simulink model "kamerol"  (R2021b)
settings: Solver=VariableStepAuto  StartTime=0.0  StopTime=10.0  RelTol=1e-3
undefined symbols (not defined in the file): admireDB
libraries: simulink_extras x104, simulink x24, sharedutil x1
(part 1 of 14)
settings Model: Creator=mehme  LastModifiedBy=mehme

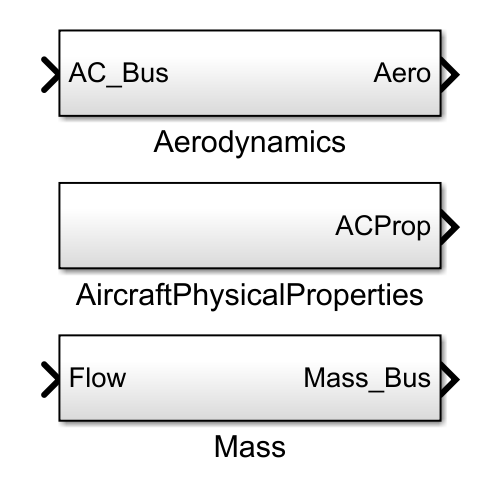
[thumbnail: Simulink's stored preview of the top-level diagram]
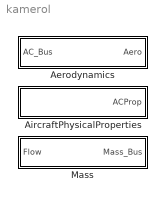
== system kamerol ==
  Aerodynamics : Subsystem
  AircraftPhysicalProperties : Subsystem
  Mass : Subsystem

== system kamerol/Aerodynamics ==
  AC_Bus : Inport
  Bus Creator1 : BusCreator  Inputs=12
  CentripetalForceCoefficient : Subsystem
  Interface : Subsystem
  NormalForceCoefficient : Subsystem
  PitchMomentCoefficient : Subsystem
  RollMomentCoefficient : Subsystem
  Subsystem : Subsystem
  TangentialForceCoefficient : Subsystem
  YawMomentCoefficient : Subsystem
  Aero : Outport
  wires:
  AC_Bus/1 -> Subsystem/7(AC_Bus), Interface/1(AC_Bus)  "AeroIn_Bus"
  PitchMomentCoefficient/1(Cpmtot) -> Subsystem/5(cpm), Bus Creator1/5  "pitchMomentCoeff_nd"
  NormalForceCoefficient/1(Cntot) -> Subsystem/3(cn), Bus Creator1/3  "normalForceCoeff_nd"
  TangentialForceCoefficient/1(Cttot) -> Bus Creator1/1, Subsystem/1(ct)  "tangentialForceCoeff_nd"
  Bus Creator1/1 -> Aero/1  "Aero_Bus"
  Interface/1(AeroIn_Bus) -> TangentialForceCoefficient/1(AeroIn_Bus), CentripetalForceCoefficient/1(AeroIn_Bus), NormalForceCoefficient/1(AeroIn_Bus), RollMomentCoefficient/1(AeroIn_Bus), YawMomentCoefficient/1(AeroIn_Bus), PitchMomentCoefficient/1(AeroIn_Bus)  "AeroIn_Bus"
  Subsystem/1(aeroForceBodyX_N) -> Bus Creator1/7  "aeroForceBodyX_N"
  Subsystem/2(aeroForceBodyY_N) -> Bus Creator1/8  "aeroForceBodyY_N"
  Subsystem/3(aeroForceBodyZ_N) -> Bus Creator1/9  "aeroForceBodyZ_N"
  Subsystem/4(aeroMomentBodyX_N) -> Bus Creator1/10  "aeroMomentBodyX_N"
  Subsystem/5(aeroMomentBodyY_N) -> Bus Creator1/11  "aeroMomentBodyY_N"
  Subsystem/6(aeroMomentBodyZ_N) -> Bus Creator1/12  "aeroMomentBodyZ_N"
  CentripetalForceCoefficient/1(Cctot) -> Subsystem/2(cc), Bus Creator1/2  "centripetalForceCoeff_nd"
  RollMomentCoefficient/1(Crmtot) -> Subsystem/4(crm), Bus Creator1/4  "rollMomentCoeff_nd"
  YawMomentCoefficient/1(Cymtot) -> Subsystem/6(cym), Bus Creator1/6  "yawMomentCoeff_nd"

== system kamerol/AircraftPhysicalProperties ==
  Bus Creator : BusCreator  Inputs=19
  EngineOffsetY_m : Constant  Value=0
  EngineOffsetZ_m : Constant  Value=-0.15
  ReferenceAreaCanard_m2 : Constant  Value=3.20
  ReferenceAreaInboardElevon_m2 : Constant  Value=1.2
  ReferenceAreaInboardLEF_m2 : Constant  Value=0.45
  ReferenceAreaOutboardElevon_m2 : Constant  Value=1.35
  ReferenceAreaOutboardLEF_m : Constant  Value=0.45
  ReferenceAreaRudder_m2 : Constant  Value=0.80
  ReferenceArea_m2 : Constant  Value=45
  ReferenceChordCanard_m : Constant  Value=1.30
  ReferenceChordInboardElevon_m : Constant  Value=0.95
  ReferenceChordInboardLEF_m : Constant  Value=0.40
  ReferenceChordOutboardElevon_m : Constant  Value=0.68
  ReferenceChordOutboardLEF_m : Constant  Value=0.35
  ReferenceChordRudder_m : Constant  Value=0.60
  ReferenceChord_m : Constant  Value=5.2
  ReferenceLengthAirbrake_m : Constant  Value=1.10
  ReferenceSpanCanard_m : Constant  Value=2.60
  ReferenceSpan_m : Constant  Value=10
  ACProp : Outport
  wires:
  ReferenceArea_m2/1 -> Bus Creator/1  "referenceArea_m2"
  ReferenceChord_m/1 -> Bus Creator/2  "referenceChord_m"
  ReferenceSpan_m/1 -> Bus Creator/3  "referenceSpan_m"
  ReferenceAreaInboardElevon_m2/1 -> Bus Creator/4  "referenceAreaInboardElevon_m2"
  ReferenceChordInboardElevon_m/1 -> Bus Creator/5  "referenceChordInboardElevon_m"
  ReferenceAreaOutboardElevon_m2/1 -> Bus Creator/6  "referenceAreaOutboardElevon_m2"
  ReferenceChordOutboardElevon_m/1 -> Bus Creator/7  "referenceChordOutboardElevon_m"
  ReferenceAreaInboardLEF_m2/1 -> Bus Creator/8  "referenceAreaInboardLEF_m2"
  ReferenceChordInboardLEF_m/1 -> Bus Creator/9  "referenceChordInboardLEF_m"
  ReferenceAreaOutboardLEF_m/1 -> Bus Creator/10  "referenceAreaOutboardLEF_m"
  ReferenceChordOutboardLEF_m/1 -> Bus Creator/11  "referenceChordOutboardLEF_m"
  ReferenceAreaRudder_m2/1 -> Bus Creator/12  "referenceAreaRudder_m2"
  ReferenceChordRudder_m/1 -> Bus Creator/13  "referenceChordRudder_m"
  ReferenceLengthAirbrake_m/1 -> Bus Creator/14  "referenceLengthAirbrake_m"
  ReferenceAreaCanard_m2/1 -> Bus Creator/15  "referenceAreaCanard_m2"
  ReferenceChordCanard_m/1 -> Bus Creator/16  "referenceChordCanard_m"
  ReferenceSpanCanard_m/1 -> Bus Creator/17  "referenceSpanCanard_m"
  Bus Creator/1 -> ACProp/1  "AC_Bus"
  EngineOffsetY_m/1 -> Bus Creator/18  "engineOffsetY_m"
  EngineOffsetZ_m/1 -> Bus Creator/19  "engineOffsetZ_m"

== system kamerol/Mass ==
  Flow : Inport
  Bus Creator1 : BusCreator  Inputs=12
  Bus Selector : BusSelector  OutputSignals=DCM_Bus.dcmNED2Body
  Constant : Constant  Value=9.8065
  Constant1 : Constant  Value=0
  Constant3 : Constant  Value=0
  Demux : Demux  Outputs=3
  Inertia : Subsystem
  Matrix Multiply : Product  Multiplication=Matrix(*)
  Mux : Mux  Inputs=3
  Product : Product
  "mass " : Constant  Value=9100
  Mass_Bus : Outport
  wires:
  Bus Creator1/1 -> Mass_Bus/1  "MassBuss"
  Demux/1 -> Bus Creator1/8  "gravForceBodyX_N"
  Demux/2 -> Bus Creator1/9  "gravForceBodyY_N"
  Demux/3 -> Bus Creator1/10  "gravForceBodyZ_N"
  Constant3/1 -> Bus Creator1/11  "centerOfGravityBodyX_pct"
  "mass "/1 -> Bus Creator1/12, Product/2  "mass_kg"
  Flow/1 -> Bus Selector/1
  Constant/1 -> Product/1
  Bus Selector/1 -> Matrix Multiply/1  "<dcmNED2Body>"
  Constant1/1 -> Mux/2, Mux/1
  Product/1 -> Mux/3
  Matrix Multiply/1 -> Demux/1
  Mux/1 -> Matrix Multiply/2
  Inertia/1(InertiaTensor) -> Bus Creator1/1
  Inertia/2(inertiaIx_kgpm2) -> Bus Creator1/2
  Inertia/3(inertiaIy_kgpm2) -> Bus Creator1/3
  Inertia/4(inertiaIz_kgpm2) -> Bus Creator1/4
  Inertia/5(inertiaIxy_kgpm2) -> Bus Creator1/5
  Inertia/6(inertiaIxz_kgpm2) -> Bus Creator1/6
  Inertia/7(inertiaIyz_kgpm2) -> Bus Creator1/7

== system kamerol/Aerodynamics/CentripetalForceCoefficient ==
  AeroIn_Bus : Inport
  Bus Selector : BusSelector  OutputSignals=mach_nd
  MachRegion1 : Subsystem
  MachRegion2 : Subsystem
  MachRegion3 : Subsystem
  MachRegion4 : Subsystem
  Subsystem : Subsystem
  Cctot : Outport
  wires:
  Subsystem/1(Cctot) -> Cctot/1
  MachRegion3/1(cctot) -> Subsystem/4(CctotMR3)
  MachRegion2/1(cctot) -> Subsystem/3(CctotMR2)
  MachRegion4/1(cttot) -> Subsystem/5(CctotMR4)
  Bus Selector/1 -> Subsystem/1(mach_nd)  "<mach_nd>"
  AeroIn_Bus/1 -> MachRegion2/1(AeroIn_Bus), MachRegion3/1(AeroIn_Bus), MachRegion4/1(AeroIn_Bus), MachRegion1/1(AeroIn_Bus), Bus Selector/1
  MachRegion1/1(cctot) -> Subsystem/2(CctotMR1)

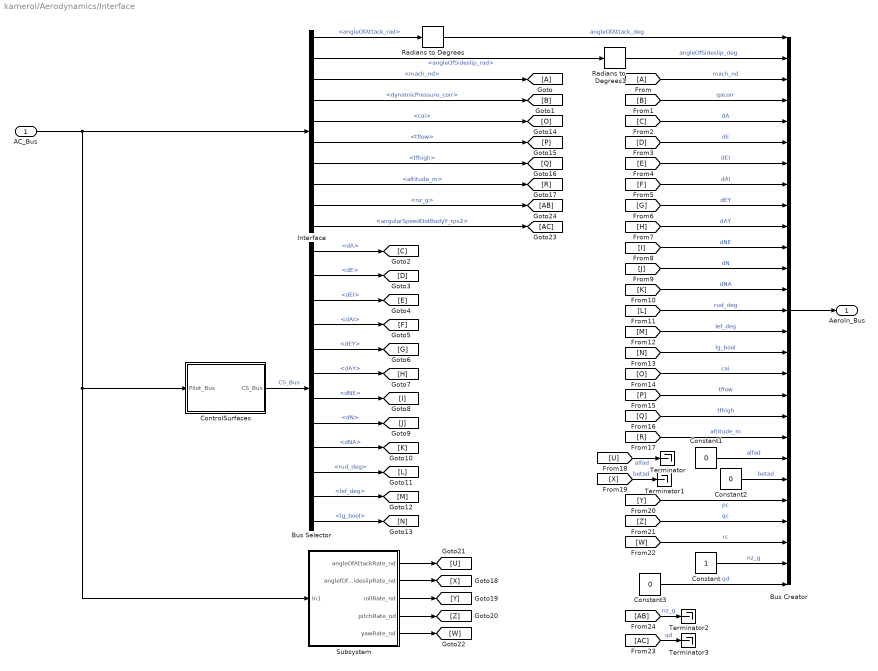
== system kamerol/Aerodynamics/Interface ==
  AC_Bus : Inport
  Bus Creator : BusCreator  Inputs=27
  Bus Selector : BusSelector  OutputSignals=dA,dE,dEI,dAI,dEY,dAY,dNE,dN,dNA,rud_deg,lef_deg,lg_bool
  Constant : Constant
  Constant1 : Constant  Value=0
  Constant2 : Constant  Value=0
  Constant3 : Constant  Value=0
  ControlSurfaces : Subsystem
  Interface : BusSelector  OutputSignals=EOM_Bus.angleOfAttack_rad,EOM_Bus.angleOfSideslip_rad,Env_Bus.mach_nd,Env_Bus.dynamicPressure_corr,Misc_Bus.cai,Env_Bus.tflow,Env_Bus.tfhigh,EOM_Bus.altitude_m,EOM_Bus.nz_g,EOM_Bus.angularSpeedDotBodyY_rps2
  Radians to Degrees : simulink_extras/Transformations/Radians to Degrees
  Radians to Degrees1 : simulink_extras/Transformations/Radians to Degrees
  Subsystem : Subsystem
  Terminator{,1..3} (4 alike) : Terminator
  AeroIn_Bus : Outport
  wires:
  AC_Bus/1 -> Subsystem/1(In1), ControlSurfaces/1(Pilot_Bus), Interface/1
  Bus Creator/1 -> AeroIn_Bus/1
  Interface/1 -> Radians to Degrees/1  "<angleOfAttack_rad>"
  Interface/2 -> Radians to Degrees1/1  "<angleOfSideslip_rad>"
  Radians to Degrees/1 -> Bus Creator/1  "angleOfAttack_deg"
  Radians to Degrees1/1 -> Bus Creator/2  "angleOfSideslip_deg"
  Interface/3 -> [A]  "<mach_nd>"
  [A] -> Bus Creator/3  "mach_nd"
  [B] -> Bus Creator/4  "qacorr"
  Interface/4 -> [B]  "<dynamicPressure_corr>"
  Interface/5 -> [O]  "<cai>"
  Interface/6 -> [P]  "<tflow>"
  Interface/7 -> [Q]  "<tfhigh>"
  Interface/8 -> [R]  "<altitude_m>"
  [C] -> Bus Creator/5  "dA"
  [D] -> Bus Creator/6  "dE"
  [E] -> Bus Creator/7  "dEI"
  [N] -> Bus Creator/16  "lg_bool"
  [F] -> Bus Creator/8  "dAI"
  [R] -> Bus Creator/20  "altitude_m"
  [O] -> Bus Creator/17  "cai"
  Constant1/1 -> Bus Creator/21  "alfad"
  Constant2/1 -> Bus Creator/22  "betad"
  [G] -> Bus Creator/9  "dEY"
  [H] -> Bus Creator/10  "dAY"
  [K] -> Bus Creator/13  "dNA"
  [L] -> Bus Creator/14  "rud_deg"
  [I] -> Bus Creator/11  "dNE"
  [J] -> Bus Creator/12  "dN"
  [M] -> Bus Creator/15  "lef_deg"
  [W] -> Bus Creator/25  "rc"
  [Q] -> Bus Creator/19  "tfhigh"
  [P] -> Bus Creator/18  "tflow"
  [Y] -> Bus Creator/23  "pc"
  [Z] -> Bus Creator/24  "qc"
  Constant/1 -> Bus Creator/26  "nz_g"
  Interface/9 -> [AB]  "<nz_g>"
  Interface/10 -> [AC]  "<angularSpeedDotBodyY_rps2>"
  Constant3/1 -> Bus Creator/27  "qd"
  Subsystem/2(anglefOfSideslipRate_nd) -> [X]
  Subsystem/1(angleOfAttackRate_nd) -> [U]
  Subsystem/3(rollRate_nd) -> [Y]
  Subsystem/4(pitchRate_nd) -> [Z]
  Subsystem/5(yawRate_nd) -> [W]
  [U] -> Terminator/1  "alfad"
  [X] -> Terminator1/1  "betad"
  [AB] -> Terminator2/1  "nz_g"
  [AC] -> Terminator3/1  "qd"
  ControlSurfaces/1(CS_Bus) -> Bus Selector/1  "CS_Bus"
  Bus Selector/1 -> [C]  "<dA>"
  Bus Selector/2 -> [D]  "<dE>"
  Bus Selector/3 -> [E]  "<dEI>"
  Bus Selector/4 -> [F]  "<dAI>"
  Bus Selector/5 -> [G]  "<dEY>"
  Bus Selector/6 -> [H]  "<dAY>"
  Bus Selector/7 -> [I]  "<dNE>"
  Bus Selector/8 -> [J]  "<dN>"
  Bus Selector/9 -> [K]  "<dNA>"
  Bus Selector/10 -> [L]  "<rud_deg>"
  Bus Selector/11 -> [M]  "<lef_deg>"
  Bus Selector/12 -> [N]  "<lg_bool>"

== system kamerol/Aerodynamics/NormalForceCoefficient ==
  AeroIn_Bus : Inport
  Bus Selector : BusSelector  OutputSignals=mach_nd
  MachRegion1 : Subsystem
  MachRegion2 : Subsystem
  MachRegion3 : Subsystem
  Subsystem : Subsystem
  Cntot : Outport
  wires:
  Subsystem/1(Cntot) -> Cntot/1
  Bus Selector/1 -> Subsystem/1(mach_nd)  "<mach_nd>"
  MachRegion2/1(Cntot) -> Subsystem/3(CntotMR2)
  AeroIn_Bus/1 -> MachRegion2/1(Misc_Bus), MachRegion3/1(Misc_Bus), MachRegion1/1(Misc_Bus), Bus Selector/1
  MachRegion3/1(Cntot) -> Subsystem/4(CntotMR3)
  MachRegion1/1(Cntot) -> Subsystem/2(CntotMR1)

== system kamerol/Aerodynamics/PitchMomentCoefficient ==
  AeroIn_Bus : Inport
  Bus Selector : BusSelector  OutputSignals=mach_nd
  MachRegion1 : Subsystem
  MachRegion2 : Subsystem
  MachRegion3 : Subsystem
  Subsystem : Subsystem
  Cpmtot : Outport
  wires:
  Subsystem/1(Cpmtot) -> Cpmtot/1
  MachRegion1/1(Cpmtot) -> Subsystem/2(CpmtotMR1)
  MachRegion2/1(Cpmtot) -> Subsystem/3(CpmtotMR2)
  MachRegion3/1(Cpmtot) -> Subsystem/4(CpmtotMR3)
  AeroIn_Bus/1 -> MachRegion2/1(Misc_Bus), MachRegion3/1(Misc_Bus), MachRegion1/1(Misc_Bus), Bus Selector/1
  Bus Selector/1 -> Subsystem/1(mach_nd)  "<mach_nd>"

== system kamerol/Aerodynamics/RollMomentCoefficient ==
  AeroIn_Bus : Inport
  Bus Selector : BusSelector  OutputSignals=mach_nd
  MachRegion1 : Subsystem
  MachRegion2 : Subsystem
  MachRegion3 : Subsystem
  MachRegion4 : Subsystem
  Subsystem : Subsystem
  Crmtot : Outport
  wires:
  Subsystem/1(Crmtot) -> Crmtot/1
  MachRegion4/1(crmtot) -> Subsystem/5(CrmtotMR4)
  MachRegion3/1(crmtot) -> Subsystem/4(CrmtotMR3)
  MachRegion2/1(crmtot) -> Subsystem/3(CrmtotMR2)
  MachRegion1/1(crmtot) -> Subsystem/2(CrmtotMR1)
  Bus Selector/1 -> Subsystem/1(mach_nd)  "<mach_nd>"
  AeroIn_Bus/1 -> MachRegion1/1(AeroIn_Bus), Bus Selector/1, MachRegion2/1(AeroIn_Bus), MachRegion3/1(AeroIn_Bus), MachRegion4/1(AeroIn_Bus)

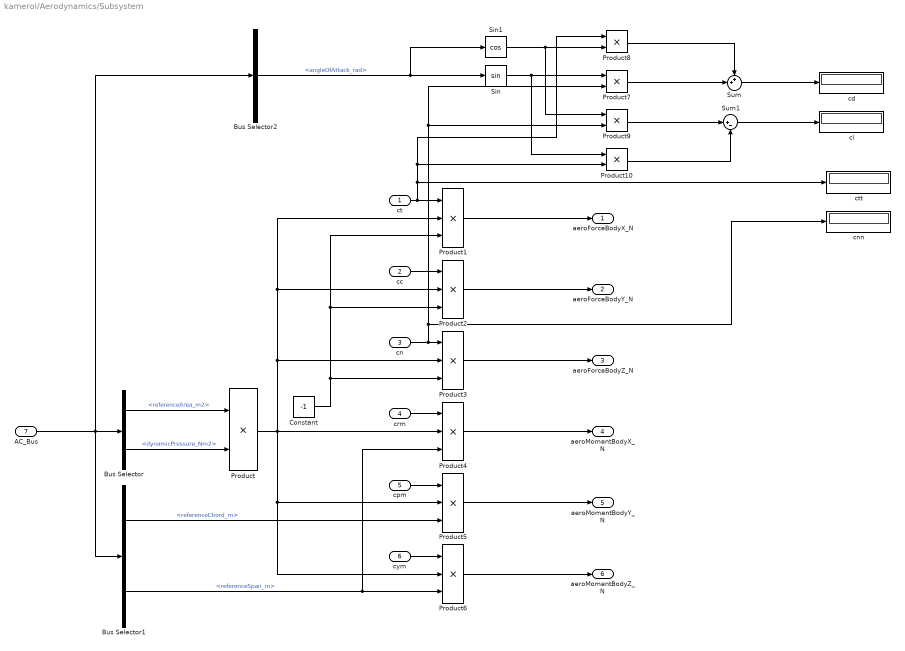
== system kamerol/Aerodynamics/Subsystem ==
  ct : Inport
  cc : Inport  Port=2
  cn : Inport  Port=3
  crm : Inport  Port=4
  cpm : Inport  Port=5
  cym : Inport  Port=6
  AC_Bus : Inport  Port=7
  Bus Selector : BusSelector  OutputSignals=AC_Bus.referenceArea_m2,Env_Bus.dynamicPressure_Nm2
  Bus Selector1 : BusSelector  OutputSignals=AC_Bus.referenceChord_m,AC_Bus.referenceSpan_m
  Bus Selector2 : BusSelector  OutputSignals=EOM_Bus.angleOfAttack_rad
  Constant : Constant  Value=-1
  Product{,7..10} (5 alike) : Product
  Product{1..6} (6 alike) : Product  Inputs=3
  Sin : Trigonometry
  Sin1 : Trigonometry  Operator=cos
  Sum : Sum  Inputs=++|
  Sum1 : Sum  Inputs=|+-
  cd : Display
  cl : Display
  cnn : Display
  ctt : Display
  aeroForceBodyX_N : Outport
  aeroForceBodyY_N : Outport  Port=2
  aeroForceBodyZ_N : Outport  Port=3
  aeroMomentBodyX_N : Outport  Port=4
  aeroMomentBodyY_N : Outport  Port=5
  aeroMomentBodyZ_N : Outport  Port=6
  wires:
  AC_Bus/1 -> Bus Selector2/1, Bus Selector1/1, Bus Selector/1
  Bus Selector/1 -> Product/1  "<referenceArea_m2>"
  Bus Selector/2 -> Product/2  "<dynamicPressure_Nm2>"
  Product/1 -> Product6/2, Product5/2, Product4/2, Product3/2, Product2/2, Product1/2
  Constant/1 -> Product3/3, Product2/3, Product1/3
  Product3/1 -> aeroForceBodyZ_N/1
  Product2/1 -> aeroForceBodyY_N/1
  Bus Selector1/1 -> Product5/3  "<referenceChord_m>"
  Bus Selector1/2 -> Product4/3, Product6/3  "<referenceSpan_m>"
  Product6/1 -> aeroMomentBodyZ_N/1
  Product5/1 -> aeroMomentBodyY_N/1
  Product4/1 -> aeroMomentBodyX_N/1
  Product1/1 -> aeroForceBodyX_N/1
  cym/1 -> Product6/1
  cpm/1 -> Product5/1
  crm/1 -> Product4/1
  ct/1 -> Product10/2, Product8/1, ctt/1, Product1/1
  cc/1 -> Product2/1
  cn/1 -> cnn/1, Product9/2, Product7/2, Product3/1
  Bus Selector2/1 -> Sin1/1, Sin/1  "<angleOfAttack_rad>"
  Sin/1 -> Product10/1, Product7/1
  Product7/1 -> Sum/2
  Sin1/1 -> Product9/1, Product8/2
  Product8/1 -> Sum/1
  Sum/1 -> cd/1
  Product9/1 -> Sum1/1
  Product10/1 -> Sum1/2
  Sum1/1 -> cl/1

== system kamerol/Aerodynamics/TangentialForceCoefficient ==
  AeroIn_Bus : Inport
  Bus Selector : BusSelector  OutputSignals=mach_nd
  MachRegion1 : Subsystem
  MachRegion2 : Subsystem
  MachRegion3 : Subsystem
  Subsystem : Subsystem
  Cttot : Outport
  wires:
  Subsystem/1(Out1) -> Cttot/1
  MachRegion3/1(cttotMR3) -> Subsystem/4(cttotMR3)
  MachRegion2/1(cttotMR2) -> Subsystem/3(cttotMR2)
  MachRegion1/1(cttotMR1) -> Subsystem/2(cttotMR1)
  Bus Selector/1 -> Subsystem/1(mach_nd)  "<mach_nd>"
  AeroIn_Bus/1 -> MachRegion1/1(AeroIn_Bus), MachRegion2/1(AeroIn_Bus), MachRegion3/1(AeroIn_Bus), Bus Selector/1  "AeroIn_Bus"

== system kamerol/Aerodynamics/YawMomentCoefficient ==
  AeroIn_Bus : Inport
  Bus Selector : BusSelector  OutputSignals=mach_nd
  MachRegion1 : Subsystem
  MachRegion2 : Subsystem
  MachRegion3 : Subsystem
  MachRegion4 : Subsystem
  Subsystem : Subsystem
  Cymtot : Outport
  wires:
  Subsystem/1(Cymtot) -> Cymtot/1
  Bus Selector/1 -> Subsystem/1(mach_nd)  "<mach_nd>"
  MachRegion1/1(Cymtot) -> Subsystem/2(CymtotMR1)
  MachRegion3/1(Cymtot) -> Subsystem/4(CymtotMR3)
  AeroIn_Bus/1 -> MachRegion1/1(AeroIn_Bus), Bus Selector/1, MachRegion2/1(AeroIn_Bus), MachRegion3/1(AeroIn_Bus), MachRegion4/1(AeroIn_Bus)
  MachRegion4/1(Cymtot) -> Subsystem/5(CymtotMR4)
  MachRegion2/1(Cymtot) -> Subsystem/3(CymtotMR2)

== system kamerol/Mass/Inertia ==
  Create 3x3 Matrix : sharedutil/Create 3x3 Matrix  aMode=aMode
      settings: SourceProductBaseCode=AE,PW,DR,MT,UV,VE
  Gain : Gain  Gain=-1
  Gain1 : Gain  Gain=-1
  Gain2 : Gain  Gain=-1
  "Ix " : Constant  Value=21000
  Ixy : Constant  Value=0
  "Ixz " : Constant  Value=2500
  "Iy " : Constant  Value=81000
  Iyz : Constant  Value=0
  "Iz " : Constant  Value=101000
  InertiaTensor : Outport
  inertiaIx_kgpm2 : Outport  Port=2
  inertiaIy_kgpm2 : Outport  Port=3
  inertiaIz_kgpm2 : Outport  Port=4
  inertiaIxy_kgpm2 : Outport  Port=5
  inertiaIxz_kgpm2 : Outport  Port=6
  inertiaIyz_kgpm2 : Outport  Port=7
  wires:
  "Ix "/1 -> Create 3x3 Matrix/1, [Ix]
  "Iz "/1 -> [Iz], Create 3x3 Matrix/9
  Gain2/1 -> Create 3x3 Matrix/6, Create 3x3 Matrix/8
  [Iy] -> inertiaIy_kgpm2/1  "inertiaIy_kgpm2"
  "Ixz "/1 -> [Ixz], Gain1/1
  Ixy/1 -> [Ixy], Gain/1
  Create 3x3 Matrix/1 -> InertiaTensor/1  "InertiaTensor"
  [Ix] -> inertiaIx_kgpm2/1  "inertiaIx_kgpm2"
  Gain/1 -> Create 3x3 Matrix/4, Create 3x3 Matrix/2
  [Iyz] -> inertiaIyz_kgpm2/1  "inertiaIyz_kgpm2"
  Gain1/1 -> Create 3x3 Matrix/7, Create 3x3 Matrix/3
  "Iy "/1 -> [Iy], Create 3x3 Matrix/5
  Iyz/1 -> [Iyz], Gain2/1
  [Ixz] -> inertiaIxz_kgpm2/1  "inertiaIxz_kgpm2"
  [Ixy] -> inertiaIxy_kgpm2/1  "inertiaIxy_kgpm2"
  [Iz] -> inertiaIz_kgpm2/1  "inertiaIz_kgpm2"

== system kamerol/Aerodynamics/CentripetalForceCoefficient/MachRegion1 ==
  note: Mach <= 0.4
  AeroIn_Bus : Inport
  Bus Creator : BusCreator  Inputs=3
  Ccbcai : Subsystem
  Ccbde : Subsystem
  Ccbdle : Subsystem
  Ccbdn : Subsystem
  Ccbeta : Subsystem
  Ccbetad : Subsystem
  Ccblg : Subsystem
  Ccdai : Subsystem
  Ccdaib : Subsystem
  Ccday : Subsystem
  Ccdayb : Subsystem
  Ccdna : Subsystem
  Ccdr : Subsystem
  Ccp : Subsystem
  Ccpbeta : Subsystem
  Ccr : Subsystem
  Ccrbeta : Subsystem
  Sum : Sum  Inputs=17
  eoeff1 : Subsystem
  cctot : Outport
  wires:
  Ccrbeta/1(Ccrbeta) -> Sum/17  "Ccrbeta"
  Ccr/1(Ccr) -> Sum/16  "Ccr"
  Ccpbeta/1(Ccpbeta) -> Sum/15  "Ccpbeta"
  Ccp/1(Ccp) -> Sum/14  "Ccp"
  Ccbetad/1(Ccbetad) -> Sum/13  "Ccbetad"
  Ccdna/1(Ccdna) -> Sum/12  "Ccdna"
  Ccdayb/1(Ccdayb) -> Sum/11  "Ccdayb"
  Ccday/1(Ccday) -> Sum/10  "Ccday"
  Ccdaib/1(Ccdaib) -> Sum/9  "Ccdaib"
  Ccdai/1(Ccdai) -> Sum/8  "Ccdai"
  Ccdr/1(Ccdr) -> Sum/7  "Ccdr"
  Ccbcai/1(Ccbcai) -> Sum/6  "Ccbcai"
  Ccbdle/1(Ccbdle) -> Sum/5  "Ccbdle"
  Ccbdn/1(Ccbdn) -> Sum/4  "Ccbdn"
  Ccbde/1(Ccbde) -> Sum/3  "Ccbde"
  Ccblg/1(Ccblg) -> Sum/2  "Ccblg"
  Ccbeta/1(Ccbeta) -> Sum/1  "Ccbeta"
  Bus Creator/1 -> Ccp/1(in_bus), Ccpbeta/1(in_bus), Ccr/1(in_bus), Ccrbeta/1(in_bus), Ccbetad/1(in_bus), Ccdna/1(in_bus), Ccdayb/1(in_bus), Ccday/1(in_bus), Ccdaib/1(in_bus), Ccdai/1(in_bus), Ccdr/1(in_bus), Ccbcai/1(in_bus), Ccbdle/1(in_bus), Ccbdn/1(in_bus), Ccbde/1(in_bus), Ccblg/1(in_bus), Ccbeta/1(in_bus)  "in_bus"
  eoeff1/2(eieff) -> Bus Creator/3  "eieff"
  AeroIn_Bus/1 -> eoeff1/1(AeroIn_Bus), Bus Creator/1
  eoeff1/1(eoeff) -> Bus Creator/2  "eoeff"
  Sum/1 -> cctot/1

== system kamerol/Aerodynamics/CentripetalForceCoefficient/MachRegion2 ==
  note: 0.4 < Mach < 0.5
  AeroIn_Bus : Inport
  Bus Creator : BusCreator  Inputs=3
  Ccbcai : Subsystem
  Ccbde : Subsystem
  Ccbdle : Subsystem
  Ccbdn : Subsystem
  Ccbeta : Subsystem
  Ccbetad : Subsystem
  Ccblg : Subsystem
  Ccdai : Subsystem
  Ccdaib : Subsystem
  Ccday : Subsystem
  Ccdayb : Subsystem
  Ccdna : Subsystem
  Ccdr : Subsystem
  Ccp : Subsystem
  Ccpbeta : Subsystem
  Ccr : Subsystem
  Ccrbeta : Subsystem
  Sum : Sum  Inputs=17
  eoeff1 : Subsystem
  cctot : Outport
  wires:
  Ccrbeta/1(Ccrbeta) -> Sum/17  "Ccrbeta"
  Ccr/1(Ccr) -> Sum/16  "Ccr"
  Ccpbeta/1(Ccpbeta) -> Sum/15  "Ccpbeta"
  Ccp/1(Ccp) -> Sum/14  "Ccp"
  Ccbetad/1(Ccbetad) -> Sum/13  "Ccbetad"
  Ccdna/1(Ccdna) -> Sum/12  "Ccdna"
  Ccdayb/1(Ccdayb) -> Sum/11  "Ccdayb"
  Ccday/1(Ccday) -> Sum/10  "Ccday"
  Ccdaib/1(Ccdaib) -> Sum/9  "Ccdaib"
  Ccdai/1(Ccdai) -> Sum/8  "Ccdai"
  Ccdr/1(Ccdr) -> Sum/7  "Ccdr"
  Ccbcai/1(Ccbcai) -> Sum/6  "Ccbcai"
  Ccbdle/1(Ccbdle) -> Sum/5  "Ccbdle"
  Ccbdn/1(Ccbdn) -> Sum/4  "Ccbdn"
  Ccbde/1(Ccbde) -> Sum/3  "Ccbde"
  Ccblg/1(Ccblg) -> Sum/2  "Ccblg"
  Ccbeta/1(Ccbeta) -> Sum/1  "Ccbeta"
  Bus Creator/1 -> Ccr/1(in_bus), Ccrbeta/1(in_bus), Ccpbeta/1(in_bus), Ccp/1(in_bus), Ccbetad/1(in_bus), Ccdna/1(in_bus), Ccdayb/1(in_bus), Ccday/1(in_bus), Ccdaib/1(in_bus), Ccdai/1(in_bus), Ccdr/1(in_bus), Ccbcai/1(in_bus), Ccbdle/1(in_bus), Ccbdn/1(in_bus), Ccbde/1(in_bus), Ccblg/1(in_bus), Ccbeta/1(in_bus)  "in_bus"
  eoeff1/1(eoeff) -> Bus Creator/2  "eoeff"
  eoeff1/2(eieff) -> Bus Creator/3  "eieff"
  AeroIn_Bus/1 -> eoeff1/1(AeroIn_Bus), Bus Creator/1
  Sum/1 -> cctot/1

== system kamerol/Aerodynamics/CentripetalForceCoefficient/MachRegion3 ==
  note: 0.5 <= Mach <= 1.4
  AeroIn_Bus : Inport
  Bus Creator : BusCreator  Inputs=3
  Ccbcai : Subsystem
  Ccbde : Subsystem
  Ccbdle : Subsystem
  Ccbdn : Subsystem
  Ccbeta : Subsystem
  Ccbetad : Subsystem
  Ccblg : Subsystem
  Ccdai : Subsystem
  Ccdaib : Subsystem
  Ccday : Subsystem
  Ccdayb : Subsystem
  Ccdna : Subsystem
  Ccdr : Subsystem
  Ccp1 : Subsystem
  Ccpbeta : Subsystem
  Ccr1 : Subsystem
  Ccrbeta : Subsystem
  Sum : Sum  Inputs=17
  eoeff1 : Subsystem
  cctot : Outport
  wires:
  Ccrbeta/1(Ccrbeta) -> Sum/17  "Ccrbeta"
  Ccr1/1(Ccr) -> Sum/16  "Ccr"
  Ccpbeta/1(Ccpbeta) -> Sum/15  "Ccpbeta"
  Ccp1/1(Ccp) -> Sum/14  "Ccp"
  Ccbetad/1(Ccbetad) -> Sum/13  "Ccbetad"
  Ccdna/1(Ccdna) -> Sum/12  "Ccdna"
  Ccdayb/1(Ccdayb) -> Sum/11  "Ccdayb"
  Ccday/1(Ccday) -> Sum/10  "Ccday"
  Ccdaib/1(Ccdaib) -> Sum/9  "Ccdaib"
  Ccdai/1(Ccdai) -> Sum/8  "Ccdai"
  Ccdr/1(Ccdr) -> Sum/7  "Ccdr"
  Ccbcai/1(Ccbcai) -> Sum/6  "Ccbcai"
  Ccbdle/1(Ccbdle) -> Sum/5  "Ccbdle"
  Ccbdn/1(Ccbdn) -> Sum/4  "Ccbdn"
  Ccbde/1(Ccbde) -> Sum/3  "Ccbde"
  Ccblg/1(Ccblg) -> Sum/2  "Ccblg"
  Ccbeta/1(Ccbeta) -> Sum/1  "Ccbeta"
  eoeff1/2(eieff) -> Bus Creator/3  "eieff"
  eoeff1/1(eoeff) -> Bus Creator/2  "eoeff"
  Bus Creator/1 -> Ccr1/1(in_bus), Ccp1/1(in_bus), Ccbetad/1(in_bus), Ccdna/1(in_bus), Ccday/1(in_bus), Ccdai/1(in_bus), Ccdr/1(in_bus), Ccbcai/1(in_bus), Ccbdle/1(in_bus), Ccbdn/1(in_bus), Ccbde/1(in_bus), Ccblg/1(in_bus), Ccbeta/1(in_bus)  "in_bus"
  AeroIn_Bus/1 -> eoeff1/1(AeroIn_Bus), Bus Creator/1
  Sum/1 -> cctot/1

== system kamerol/Aerodynamics/CentripetalForceCoefficient/MachRegion4 ==
  note: 1.4 < Mach
  AeroIn_Bus : Inport
  Bus Creator : BusCreator  Inputs=3
  Ccbcai : Subsystem
  Ccbde : Subsystem
  Ccbdle : Subsystem
  Ccbdn : Subsystem
  Ccbeta : Subsystem
  Ccbetad : Subsystem
  Ccblg : Subsystem
  Ccdai : Subsystem
  Ccdaib : Subsystem
  Ccday : Subsystem
  Ccdayb : Subsystem
  Ccdna : Subsystem
  Ccdr : Subsystem
  Ccp : Subsystem
  Ccpbeta : Subsystem
  Ccr : Subsystem
  Ccrbeta : Subsystem
  Sum : Sum  Inputs=17
  eoeff : Subsystem
  cttot : Outport
  wires:
  Ccrbeta/1(Ccrbeta) -> Sum/17  "Ccrbeta"
  Ccr/1(Ccr) -> Sum/16  "Ccr"
  Ccpbeta/1(Ccpbeta) -> Sum/15  "Ccpbeta"
  Ccp/1(Ccp) -> Sum/14  "Ccp"
  Ccbetad/1(Ccbetad) -> Sum/13  "Ccbetad"
  Ccdna/1(Ccdna) -> Sum/12  "Ccdna"
  Ccdayb/1(Ccdayb) -> Sum/11  "Ccdayb"
  Ccday/1(Ccday) -> Sum/10  "Ccday"
  Ccdaib/1(Ccdaib) -> Sum/9  "Ccdaib"
  Ccdai/1(Ccdai) -> Sum/8  "Ccdai"
  Ccblg/1(Ccblg) -> Sum/7  "Ccblg"
  Ccdr/1(Ccdr) -> Sum/6  "Ccdr"
  Ccbcai/1(Ccbcai) -> Sum/5  "Ccbcai"
  Ccbdle/1(Ccbdle) -> Sum/4  "Ccbdle"
  Ccbdn/1(Ccbdn) -> Sum/3  "Ccbdn"
  Ccbde/1(Ccbde) -> Sum/2  "Ccbde"
  Ccbeta/1(Ccbeta) -> Sum/1  "Ccbeta"
  AeroIn_Bus/1 -> eoeff/1(AeroIn_Bus), Bus Creator/1
  Bus Creator/1 -> Ccbde/1(in_bus), Ccbdn/1(in_bus), Ccbdle/1(in_bus), Ccbcai/1(in_bus), Ccdr/1(in_bus), Ccr/1(in_bus), Ccp/1(in_bus), Ccbetad/1(in_bus), Ccdna/1(in_bus), Ccday/1(in_bus), Ccdai/1(in_bus), Ccblg/1(in_bus), Ccbeta/1(in_bus)  "in_bus"
  eoeff/2(eieff) -> Bus Creator/3  "eieff"
  eoeff/1(eoeff) -> Bus Creator/2  "eoeff"
  Sum/1 -> cttot/1

== system kamerol/Aerodynamics/CentripetalForceCoefficient/Subsystem ==
  mach_nd : Inport
  CctotMR1 : Inport  Port=2
  CctotMR2 : Inport  Port=3
  CctotMR3 : Inport  Port=4
  CctotMR4 : Inport  Port=5
  AND : Logic  IconShape=distinctive  AllPortsSameDT=off  OutDataTypeStr=boolean
  AND1 : Logic  IconShape=distinctive  AllPortsSameDT=off  OutDataTypeStr=boolean
  Compare To Constant1 : simulink/Logic and Bit Operations/Compare To Constant  relop=<=  const=0.4  OutDataTypeStr=boolean
  Compare To Constant2 : simulink/Logic and Bit Operations/Compare To Constant  relop=>  const=0.4  OutDataTypeStr=boolean
  Compare To Constant3 : simulink/Logic and Bit Operations/Compare To Constant  relop=<  const=0.5  OutDataTypeStr=boolean
  Compare To Constant4 : simulink/Logic and Bit Operations/Compare To Constant  relop=<=  const=1.4  OutDataTypeStr=boolean
  Compare To Constant5 : simulink/Logic and Bit Operations/Compare To Constant  relop=>=  const=0.5  OutDataTypeStr=boolean
  Switch : Switch  Criteria=u2 ~= 0
  Switch1 : Switch  Criteria=u2 ~= 0
  Switch2 : Switch  Criteria=u2 ~= 0
  Cctot : Outport
  wires:
  Switch/1 -> Cctot/1
  Compare To Constant5/1 -> AND1/1
  Compare To Constant4/1 -> AND1/2
  AND1/1 -> Switch2/2
  CctotMR4/1 -> Switch2/3
  CctotMR3/1 -> Switch2/1
  CctotMR1/1 -> Switch/1
  Switch2/1 -> Switch1/3
  CctotMR2/1 -> Switch1/1
  Switch1/1 -> Switch/3
  AND/1 -> Switch1/2
  Compare To Constant3/1 -> AND/2
  Compare To Constant2/1 -> AND/1
  Compare To Constant1/1 -> Switch/2
  mach_nd/1 -> Compare To Constant1/1, Compare To Constant3/1, Compare To Constant4/1, Compare To Constant5/1, Compare To Constant2/1

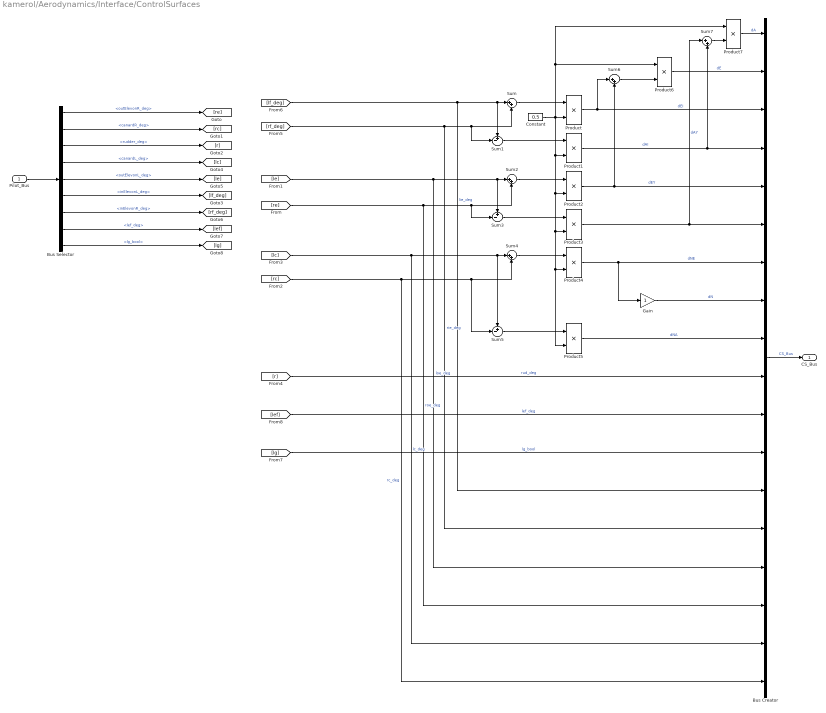
== system kamerol/Aerodynamics/Interface/ControlSurfaces ==
  Pilot_Bus : Inport
  Bus Creator : BusCreator  Inputs=18
  Bus Selector : BusSelector  OutputSignals=CS_Bus.outElevonR_deg,CS_Bus.canardR_deg,CS_Bus.rudder_deg,CS_Bus.canardL_deg,CS_Bus.outElevonL_deg,CS_Bus.inElevonL_deg,CS_Bus.inElevonR_deg,CS_Bus.lef_deg,CS_Bus.lg_bool
  Constant : Constant  Value=0.5
  Gain : Gain
  Product{,1..7} (8 alike) : Product
  Sum{,2,4,6..7} (5 alike) : Sum  Inputs=|++
  Sum1 : Sum  Inputs=+-|
  Sum3 : Sum  Inputs=+-|
  Sum5 : Sum  Inputs=+-|
  CS_Bus : Outport
  wires:
  Product/1 -> Sum6/1, Bus Creator/3  "dEI"
  [lf_deg] -> Bus Creator/13, Sum1/1, Sum/1  "lie_deg"
  Product1/1 -> Sum7/2, Bus Creator/4  "dAI"
  Product2/1 -> Sum6/2, Bus Creator/5  "dEY"
  Product3/1 -> Bus Creator/6, Sum7/1  "dAY"
  Product5/1 -> Bus Creator/9  "dNA"
  Product4/1 -> Gain/1, Bus Creator/7  "dNE"
  Gain/1 -> Bus Creator/8  "dN"
  Constant/1 -> Product7/1, Product6/1, Product5/2, Product4/2, Product3/2, Product2/2, Product1/2, Product/2
  Sum6/1 -> Product6/2
  Product6/1 -> Bus Creator/2  "dE"
  Bus Creator/1 -> CS_Bus/1  "CS_Bus"
  [lg] -> Bus Creator/12  "lg_bool"
  Sum/1 -> Product/1
  Sum2/1 -> Product2/1
  Sum1/1 -> Product1/1
  Sum3/1 -> Product3/1
  Sum4/1 -> Product4/1
  Sum5/1 -> Product5/1
  Sum7/1 -> Product7/2
  Product7/1 -> Bus Creator/1  "dA"
  [rf_deg] -> Bus Creator/14, Sum1/2, Sum/2  "rie_deg"
  [le] -> Sum2/1, Sum3/1, Bus Creator/15  "loe_deg"
  [re] -> Sum3/2, Sum2/2, Bus Creator/16  "roe_deg"
  [lc] -> Sum5/1, Sum4/1, Bus Creator/17  "lc_deg"
  [rc] -> Bus Creator/18, Sum5/2, Sum4/2  "rc_deg"
  [r] -> Bus Creator/10  "rud_deg"
  [lef] -> Bus Creator/11  "lef_deg"
  Pilot_Bus/1 -> Bus Selector/1
  Bus Selector/1 -> [re]  "<outElevonR_deg>"
  Bus Selector/2 -> [rc]  "<canardR_deg>"
  Bus Selector/3 -> [r]  "<rudder_deg>"
  Bus Selector/4 -> [lc]  "<canardL_deg>"
  Bus Selector/5 -> [le]  "<outElevonL_deg>"
  Bus Selector/7 -> [rf_deg]  "<inElevonR_deg>"
  Bus Selector/6 -> [lf_deg]  "<inElevonL_deg>"
  Bus Selector/8 -> [lef]  "<lef_deg>"
  Bus Selector/9 -> [lg]  "<lg_bool>"

== system kamerol/Aerodynamics/Interface/Subsystem ==
  In1 : Inport
  Bus Selector : BusSelector  OutputSignals=AC_Bus.referenceChord_m,EOM_Bus.speedWindX_mps,AC_Bus.referenceSpan_m,EOM_Bus.angleOfAttackDot_rps2,EOM_Bus.angleOfSideslipDot_rps2,EOM_Bus.angularSpeedBodyX_rps,EOM_Bus.angularSpeedBodyY_rps,EOM_Bus.angularSpeedBodyZ_rps
  Constant : Constant  Value=2
  Constant1 : Constant  Value=0.1
  Max : MinMax  Function=max  Inputs=2
  Product : Product  Inputs=*/
  Product1 : Product  Inputs=*/
  Product2 : Product  Inputs=/*
  Product3 : Product  Inputs=/*
  Product{4..8} (5 alike) : Product
  angleOfAttackRate_nd : Outport
  anglefOfSideslipRate_nd : Outport  Port=2
  rollRate_nd : Outport  Port=3
  pitchRate_nd : Outport  Port=4
  yawRate_nd : Outport  Port=5
  wires:
  In1/1 -> Bus Selector/1
  Constant/1 -> Product3/1, Product2/1
  Product1/1 -> Product3/2
  Bus Selector/2 -> Max/2  "<speedWindX_mps>"
  Bus Selector/1 -> Product/1  "<referenceChord_m>"
  Product/1 -> Product2/2
  Bus Selector/3 -> Product1/1  "<referenceSpan_m>"
  Product7/1 -> pitchRate_nd/1  "pitchRate_nd"
  Product5/1 -> anglefOfSideslipRate_nd/1  "anglefOfSideslipRate_nd"
  Product3/1 -> Product5/2, Product6/2, Product8/2
  Product6/1 -> rollRate_nd/1  "rollRate_nd"
  Product2/1 -> Product4/2, Product7/2
  Product8/1 -> yawRate_nd/1  "yawRate_nd"
  Product4/1 -> angleOfAttackRate_nd/1  "angleOfAttackRate_nd"
  Bus Selector/4 -> Product4/1  "<angleOfAttackDot_rps2>"
  Bus Selector/5 -> Product5/1  "<angleOfSideslipDot_rps2>"
  Bus Selector/6 -> Product6/1  "<angularSpeedBodyX_rps>"
  Bus Selector/8 -> Product8/1  "<angularSpeedBodyZ_rps>"
  Bus Selector/7 -> Product7/1  "<angularSpeedBodyY_rps>"
  Max/1 -> Product1/2, Product/2
  Constant1/1 -> Max/1

== system kamerol/Aerodynamics/NormalForceCoefficient/MachRegion1 ==
  note: Mach <= 0.4
  Misc_Bus : Inport
  Bus Creator : BusCreator  Inputs=3
  Cnalfa : Subsystem
  Cnalfad : Subsystem
  Cnbasic : Subsystem
  Cnbeta : Subsystem
  Cncai : Subsystem
  Cndedn : Subsystem
  Cndei : Subsystem
  Cndey : Subsystem
  Cndle : Subsystem
  Cndn : Subsystem
  Cnhigh : Subsystem
  Cnlg : Subsystem
  Cnnz : Subsystem
  Cnq : Subsystem
  Cnqd : Subsystem
  Sum : Sum  Inputs=15
  eoeff : Subsystem
  Cntot : Outport
  wires:
  Sum/1 -> Cntot/1
  Cnhigh/1(Cnhigh) -> Sum/15  "Cnhigh"
  Cnqd/1(Cnqd) -> Sum/14  "Cnqd"
  Cnnz/1(Cnnz) -> Sum/13  "Cnnz"
  Cnq/1(Cnq) -> Sum/12  "Cnq"
  Cnalfad/1(Cnalfad) -> Sum/11  "Cnalfad"
  Cnlg/1(Cnlg) -> Sum/10  "Cnlg"
  Cnbeta/1(Cnbeta) -> Sum/9  "Cnbeta"
  Cncai/1(Cncai) -> Sum/8  "Cncai"
  Cndle/1(Cndle) -> Sum/7  "Cndle"
  Cndn/1(Cndn) -> Sum/6  "Cndn"
  Cndedn/1(Cndedn) -> Sum/5  "Cndedn"
  Cndey/1(Cndey) -> Sum/4  "Cndey"
  Cndei/1(Cndei) -> Sum/3  "Cndei"
  Cnalfa/1(Cnalfa) -> Sum/2  "Cnalfa"
  Cnbasic/1(Cnbasic) -> Sum/1  "Cnbasic"
  Bus Creator/1 -> Cnbasic/1(in_bus), Cnalfa/1(in_bus), Cndei/1(in_bus), Cndey/1(in_bus), Cndedn/1(in_bus), Cndn/1(in_bus), Cndle/1(in_bus), Cncai/1(in_bus), Cnbeta/1(in_bus), Cnlg/1(in_bus), Cnalfad/1(in_bus), Cnq/1(in_bus), Cnnz/1(in_bus), Cnqd/1(in_bus), Cnhigh/1(in_bus)  "in_bus"
  eoeff/1(eoeff) -> Bus Creator/2  "eoeff"
  Misc_Bus/1 -> eoeff/1(AeroIn_Bus), Bus Creator/1
  eoeff/2(eieff) -> Bus Creator/3  "eieff"

== system kamerol/Aerodynamics/NormalForceCoefficient/MachRegion2 ==
  note: 0.4 < Mach < 0.5
  Misc_Bus : Inport
  Bus Creator : BusCreator  Inputs=3
  Cnalfa : Subsystem
  Cnalfad : Subsystem
  Cnbasic : Subsystem
  Cnbeta : Subsystem
  Cncai : Subsystem
  Cndedn : Subsystem
  Cndei : Subsystem
  Cndey : Subsystem
  Cndle : Subsystem
  Cndn : Subsystem
  Cnhigh : Subsystem
  Cnlg : Subsystem
  Cnnz : Subsystem
  Cnq : Subsystem
  Cnqd : Subsystem
  Sum : Sum  Inputs=15
  eoeff : Subsystem
  Cntot : Outport
  wires:
  Sum/1 -> Cntot/1
  eoeff/2(eieff) -> Bus Creator/3  "eieff"
  Misc_Bus/1 -> Bus Creator/1, eoeff/1(AeroIn_Bus)
  eoeff/1(eoeff) -> Bus Creator/2  "eoeff"
  Bus Creator/1 -> Cnqd/1(in_bus), Cnnz/1(in_bus), Cnq/1(in_bus), Cnalfad/1(in_bus), Cnlg/1(in_bus), Cnbeta/1(in_bus), Cncai/1(in_bus), Cndle/1(in_bus), Cndn/1(in_bus), Cndedn/1(in_bus), Cndey/1(in_bus), Cndei/1(in_bus), Cnalfa/1(in_bus), Cnbasic/1(in_bus)  "in_bus"
  Cnbasic/1(Cnbasic) -> Sum/1  "Cnbasic"
  Cnalfa/1(Cnalfa) -> Sum/2  "Cnalfa"
  Cndei/1(Cndei) -> Sum/3  "Cndei"
  Cndey/1(Cndey) -> Sum/4  "Cndey"
  Cndedn/1(Cndedn) -> Sum/5  "Cndedn"
  Cndn/1(Cndn) -> Sum/6  "Cndn"
  Cndle/1(Cndle) -> Sum/7  "Cndle"
  Cncai/1(Cncai) -> Sum/8  "Cncai"
  Cnbeta/1(Cnbeta) -> Sum/9  "Cnbeta"
  Cnlg/1(Cnlg) -> Sum/10  "Cnlg"
  Cnalfad/1(Cnalfad) -> Sum/11  "Cnalfad"
  Cnq/1(Cnq) -> Sum/12  "Cnq"
  Cnnz/1(Cnnz) -> Sum/13  "Cnnz"
  Cnqd/1(Cnqd) -> Sum/14  "Cnqd"
  Cnhigh/1(Cnhigh) -> Sum/15  "Cnhigh"

== system kamerol/Aerodynamics/NormalForceCoefficient/MachRegion3 ==
  note: 0.5 <= Mach
  Misc_Bus : Inport
  Bus Creator : BusCreator  Inputs=3
  Cnalfa : Subsystem
  Cnalfad : Subsystem
  Cnbasic : Subsystem
  Cnbeta : Subsystem
  Cncai : Subsystem
  Cndedn : Subsystem
  Cndei : Subsystem
  Cndey : Subsystem
  Cndle : Subsystem
  Cndn : Subsystem
  Cnhigh : Subsystem
  Cnlg : Subsystem
  Cnnz : Subsystem
  Cnq : Subsystem
  Cnqd : Subsystem
  Sum : Sum  Inputs=15
  eoeff : Subsystem
  Cntot : Outport
  wires:
  Sum/1 -> Cntot/1
  eoeff/2(eieff) -> Bus Creator/3  "eieff"
  Misc_Bus/1 -> Bus Creator/1, eoeff/1(AeroIn_Bus)
  eoeff/1(eoeff) -> Bus Creator/2  "eoeff"
  Bus Creator/1 -> Cnqd/1(in_bus), Cnnz/1(in_bus), Cnq/1(in_bus), Cnalfad/1(in_bus), Cnlg/1(in_bus), Cncai/1(in_bus), Cndle/1(in_bus), Cndn/1(in_bus), Cndey/1(in_bus), Cndei/1(in_bus), Cnalfa/1(in_bus), Cnbasic/1(in_bus)  "in_bus"
  Cnbasic/1(Cnbasic) -> Sum/1  "Cnbasic"
  Cnalfa/1(Cnalfa) -> Sum/2  "Cnalfa"
  Cndei/1(Cndei) -> Sum/3  "Cndei"
  Cndey/1(Cndey) -> Sum/4  "Cndey"
  Cndedn/1(Cndedn) -> Sum/5  "Cndedn"
  Cndn/1(Cndn) -> Sum/6  "Cndn"
  Cndle/1(Cndle) -> Sum/7  "Cndle"
  Cncai/1(Cncai) -> Sum/8  "Cncai"
  Cnbeta/1(Cnbeta) -> Sum/9  "Cnbeta"
  Cnlg/1(Cnlg) -> Sum/10  "Cnlg"
  Cnalfad/1(Cnalfad) -> Sum/11  "Cnalfad"
  Cnq/1(Cnq) -> Sum/12  "Cnq"
  Cnnz/1(Cnnz) -> Sum/13  "Cnnz"
  Cnqd/1(Cnqd) -> Sum/14  "Cnqd"
  Cnhigh/1(Cnhigh) -> Sum/15  "Cnhigh"

== system kamerol/Aerodynamics/NormalForceCoefficient/Subsystem ==
  mach_nd : Inport
  CntotMR1 : Inport  Port=2
  CntotMR2 : Inport  Port=3
  CntotMR3 : Inport  Port=4
  AND : Logic  IconShape=distinctive  AllPortsSameDT=off  OutDataTypeStr=boolean
  Compare To Constant1 : simulink/Logic and Bit Operations/Compare To Constant  relop=<=  const=0.4  OutDataTypeStr=boolean
  Compare To Constant2 : simulink/Logic and Bit Operations/Compare To Constant  relop=>  const=0.4  OutDataTypeStr=boolean
  Compare To Constant3 : simulink/Logic and Bit Operations/Compare To Constant  relop=<  const=0.5  OutDataTypeStr=boolean
  Switch : Switch  Criteria=u2 ~= 0
  Switch1 : Switch  Criteria=u2 ~= 0
  Cntot : Outport
  wires:
  Switch/1 -> Cntot/1
  CntotMR3/1 -> Switch1/3
  CntotMR2/1 -> Switch1/1
  Switch1/1 -> Switch/3
  CntotMR1/1 -> Switch/1
  AND/1 -> Switch1/2
  Compare To Constant3/1 -> AND/2
  Compare To Constant2/1 -> AND/1
  Compare To Constant1/1 -> Switch/2
  mach_nd/1 -> Compare To Constant1/1, Compare To Constant3/1, Compare To Constant2/1

== system kamerol/Aerodynamics/PitchMomentCoefficient/MachRegion1 ==
  note: Mach <= 0.4
  Misc_Bus : Inport
  Bus Creator : BusCreator  Inputs=3
  Cpmalfa : Subsystem
  Cpmalfad : Subsystem
  Cpmbasic : Subsystem
  Cpmbeta : Subsystem
  Cpmcai : Subsystem
  Cpmda : Subsystem
  Cpmdedn : Subsystem
  Cpmdei : Subsystem
  Cpmdey : Subsystem
  Cpmdle : Subsystem
  Cpmdn : Subsystem
  Cpmhigh : Subsystem
  Cpmlg : Subsystem
  Cpmnz : Subsystem
  Cpmq : Subsystem
  Cpmqd : Subsystem
  Sum : Sum  Inputs=16
  eoeff : Subsystem
  Cpmtot : Outport
  wires:
  Cpmhigh/1(Cpmhigh) -> Sum/16  "Cpmhigh"
  Cpmqd/1(Cpmqd) -> Sum/15  "Cpmqd"
  Cpmnz/1(Cpmnz) -> Sum/14  "Cpmnz"
  Cpmq/1(Cpmq) -> Sum/13  "Cpmq"
  Cpmalfad/1(Cpmalfad) -> Sum/12  "Cpmalfad"
  Cpmda/1(Cpmda) -> Sum/11  "Cpmda"
  Cpmbasic/1(Cpmbasic) -> Sum/1  "Cpmbasic"
  Cpmbeta/1(Cpmbeta) -> Sum/10  "Cpmbeta"
  Cpmalfa/1(Cpmalfa) -> Sum/2  "Cpmalfa"
  Cpmcai/1(Cpmcai) -> Sum/9  "Cpmcai"
  Cpmdei/1(Cpmdei) -> Sum/3  "Cpmdei"
  Cpmlg/1(Cpmlg) -> Sum/8  "Cpmlg"
  Cpmdey/1(Cpmdey) -> Sum/4  "Cpmdey"
  Cpmdle/1(Cpmdle) -> Sum/7  "Cpmdle"
  Cpmdedn/1(Cpmdedn) -> Sum/5  "Cpmdedn"
  Cpmdn/1(Cpmdn) -> Sum/6  "Cpmdn"
  Bus Creator/1 -> Cpmbasic/1(in_bus), Cpmnz/1(in_bus), Cpmqd/1(in_bus), Cpmhigh/1(in_bus), Cpmq/1(in_bus), Cpmalfad/1(in_bus), Cpmda/1(in_bus), Cpmbeta/1(in_bus), Cpmcai/1(in_bus), Cpmlg/1(in_bus), Cpmdle/1(in_bus), Cpmdn/1(in_bus), Cpmdedn/1(in_bus), Cpmdey/1(in_bus), Cpmdei/1(in_bus), Cpmalfa/1(in_bus)  "in_bus"
  eoeff/1(eoeff) -> Bus Creator/2  "eoeff"
  eoeff/2(eieff) -> Bus Creator/3  "eieff"
  Misc_Bus/1 -> eoeff/1(AeroIn_Bus), Bus Creator/1
  Sum/1 -> Cpmtot/1

== system kamerol/Aerodynamics/PitchMomentCoefficient/MachRegion2 ==
  note: 0.4 < Mach < 0.5
  Misc_Bus : Inport
  Bus Creator : BusCreator  Inputs=5
  Cpmalfa : Subsystem
  Cpmalfad : Subsystem
  Cpmbasic : Subsystem
  Cpmbeta : Subsystem
  Cpmcai : Subsystem
  Cpmda : Subsystem
  Cpmdedn : Subsystem
  Cpmdei : Subsystem
  Cpmdey : Subsystem
  Cpmdle : Subsystem
  Cpmdn : Subsystem
  Cpmhigh : Subsystem
  Cpmlg : Subsystem
  Cpmnz : Subsystem
  Cpmq : Subsystem
  Cpmqd : Subsystem
  Sum : Sum  Inputs=16
  eoeff : Subsystem
  Cpmtot : Outport
  wires:
  eoeff/3(eoefflow) -> Bus Creator/4  "eoefflow"
  eoeff/4(eiefflow) -> Bus Creator/5  "eiefflow"
  Sum/1 -> Cpmtot/1
  Misc_Bus/1 -> Bus Creator/1, eoeff/1(AeroIn_Bus)
  eoeff/2(eieff) -> Bus Creator/3  "eieff"
  eoeff/1(eoeff) -> Bus Creator/2  "eoeff"
  Bus Creator/1 -> Cpmalfa/1(in_bus), Cpmdei/1(in_bus), Cpmdedn/1(in_bus), Cpmdn/1(in_bus), Cpmdle/1(in_bus), Cpmlg/1(in_bus), Cpmcai/1(in_bus), Cpmbeta/1(in_bus), Cpmda/1(in_bus), Cpmalfad/1(in_bus), Cpmq/1(in_bus), Cpmqd/1(in_bus), Cpmnz/1(in_bus), Cpmdey/1(in_bus), Cpmbasic/1(in_bus)  "in_bus"
  Cpmdn/1(Cpmdn) -> Sum/6  "Cpmdn"
  Cpmdedn/1(Cpmdedn) -> Sum/5  "Cpmdedn"
  Cpmdle/1(Cpmdle) -> Sum/7  "Cpmdle"
  Cpmdey/1(Cpmdey) -> Sum/4  "Cpmdey"
  Cpmlg/1(Cpmlg) -> Sum/8  "Cpmlg"
  Cpmdei/1(Cpmdei) -> Sum/3  "Cpmdei"
  Cpmcai/1(Cpmcai) -> Sum/9  "Cpmcai"
  Cpmalfa/1(Cpmalfa) -> Sum/2  "Cpmalfa"
  Cpmbeta/1(Cpmbeta) -> Sum/10  "Cpmbeta"
  Cpmbasic/1(Cpmbasic) -> Sum/1  "Cpmbasic"
  Cpmda/1(Cpmda) -> Sum/11  "Cpmda"
  Cpmalfad/1(Cpmalfad) -> Sum/12  "Cpmalfad"
  Cpmq/1(Cpmq) -> Sum/13  "Cpmq"
  Cpmnz/1(Cpmnz) -> Sum/14  "Cpmnz"
  Cpmqd/1(Cpmqd) -> Sum/15  "Cpmqd"
  Cpmhigh/1(Cpmhigh) -> Sum/16  "Cpmhigh"

== system kamerol/Aerodynamics/PitchMomentCoefficient/MachRegion3 ==
  note: 0.5 <= Mach
  Misc_Bus : Inport
  Bus Creator : BusCreator  Inputs=3
  Cpmalfa : Subsystem
  Cpmalfad : Subsystem
  Cpmbasic : Subsystem
  Cpmbeta : Subsystem
  Cpmcai : Subsystem
  Cpmda : Subsystem
  Cpmdedn : Subsystem
  Cpmdei : Subsystem
  Cpmdey : Subsystem
  Cpmdle : Subsystem
  Cpmdn : Subsystem
  Cpmhigh : Subsystem
  Cpmlg : Subsystem
  Cpmnz : Subsystem
  Cpmq : Subsystem
  Cpmqd : Subsystem
  Sum : Sum  Inputs=16
  eoeff : Subsystem
  Cpmtot : Outport
  wires:
  Sum/1 -> Cpmtot/1
  Misc_Bus/1 -> Bus Creator/1, eoeff/1(AeroIn_Bus)
  eoeff/2(eieff) -> Bus Creator/3  "eieff"
  eoeff/1(eoeff) -> Bus Creator/2  "eoeff"
  Bus Creator/1 -> Cpmalfa/1(in_bus), Cpmdei/1(in_bus), Cpmdn/1(in_bus), Cpmdle/1(in_bus), Cpmlg/1(in_bus), Cpmcai/1(in_bus), Cpmalfad/1(in_bus), Cpmq/1(in_bus), Cpmqd/1(in_bus), Cpmnz/1(in_bus), Cpmdey/1(in_bus), Cpmbasic/1(in_bus)  "in_bus"
  Cpmdn/1(Cpmdn) -> Sum/6  "Cpmdn"
  Cpmdedn/1(Cpmdedn) -> Sum/5  "Cpmdedn"
  Cpmdle/1(Cpmdle) -> Sum/7  "Cpmdle"
  Cpmdey/1(Cpmdey) -> Sum/4  "Cpmdey"
  Cpmlg/1(Cpmlg) -> Sum/8  "Cpmlg"
  Cpmdei/1(Cpmdei) -> Sum/3  "Cpmdei"
  Cpmcai/1(Cpmcai) -> Sum/9  "Cpmcai"
  Cpmalfa/1(Cpmalfa) -> Sum/2  "Cpmalfa"
  Cpmbeta/1(Cpmbeta) -> Sum/10  "Cpmbeta"
  Cpmbasic/1(Cpmbasic) -> Sum/1  "Cpmbasic"
  Cpmda/1(Cpmda) -> Sum/11  "Cpmda"
  Cpmalfad/1(Cpmalfad) -> Sum/12  "Cpmalfad"
  Cpmq/1(Cpmq) -> Sum/13  "Cpmq"
  Cpmnz/1(Cpmnz) -> Sum/14  "Cpmnz"
  Cpmqd/1(Cpmqd) -> Sum/15  "Cpmqd"
  Cpmhigh/1(Cpmhigh) -> Sum/16  "Cpmhigh"

== system kamerol/Aerodynamics/PitchMomentCoefficient/Subsystem ==
  mach_nd : Inport
  CpmtotMR1 : Inport  Port=2
  CpmtotMR2 : Inport  Port=3
  CpmtotMR3 : Inport  Port=4
  AND : Logic  IconShape=distinctive  AllPortsSameDT=off  OutDataTypeStr=boolean
  Compare To Constant1 : simulink/Logic and Bit Operations/Compare To Constant  relop=<=  const=0.4  OutDataTypeStr=boolean
  Compare To Constant2 : simulink/Logic and Bit Operations/Compare To Constant  relop=>  const=0.4  OutDataTypeStr=boolean
  Compare To Constant3 : simulink/Logic and Bit Operations/Compare To Constant  relop=<  const=0.5  OutDataTypeStr=boolean
  Switch : Switch  Criteria=u2 ~= 0
  Switch1 : Switch  Criteria=u2 ~= 0
  Cpmtot : Outport
  wires:
  Switch/1 -> Cpmtot/1
  CpmtotMR3/1 -> Switch1/3
  CpmtotMR2/1 -> Switch1/1
  Switch1/1 -> Switch/3
  CpmtotMR1/1 -> Switch/1
  AND/1 -> Switch1/2
  Compare To Constant3/1 -> AND/2
  Compare To Constant2/1 -> AND/1
  Compare To Constant1/1 -> Switch/2
  mach_nd/1 -> Compare To Constant1/1, Compare To Constant3/1, Compare To Constant2/1

== system kamerol/Aerodynamics/RollMomentCoefficient/MachRegion1 ==
  note: Mach <= 0.4
  AeroIn_Bus : Inport
  Bus Creator : BusCreator  Inputs=3
  Crmbasic : Subsystem
  Crmbde : Subsystem
  Crmbdle : Subsystem
  Crmbdn : Subsystem
  Crmbeta : Subsystem
  Crmbetad : Subsystem
  Crmblg : Subsystem
  Crmdai : Subsystem
  Crmdaib : Subsystem
  Crmday : Subsystem
  Crmdayb : Subsystem
  Crmdna : Subsystem
  Crmdr : Subsystem
  Crmp : Subsystem
  Crmpbeta : Subsystem
  Crmr : Subsystem
  Crmrbeta : Subsystem
  Crmrde : Subsystem
  Sum : Sum  Inputs=18
  eoeff1 : Subsystem
  crmtot : Outport
  wires:
  Crmrde/1(Crmrbeta) -> Sum/18  "Crmrde"
  Crmrbeta/1(Crmrbeta) -> Sum/17  "Crmrbeta"
  Crmr/1(Crmr) -> Sum/16  "Crmr"
  Crmpbeta/1(Crmpbeta) -> Sum/15  "Crmpbeta"
  Crmp/1(Crmp) -> Sum/14  "Crmp"
  Crmbetad/1(Crmbetad) -> Sum/13  "Crmbetad"
  Crmdna/1(Crmdna) -> Sum/12  "Crmdna"
  Crmdayb/1(Crmdayb) -> Sum/11  "Crmdayb"
  Crmday/1(Crmday) -> Sum/10  "Crmday"
  Crmdaib/1(Crmdaib) -> Sum/9  "Crmdaib"
  Crmdai/1(Crmdai) -> Sum/8  "Crmdai"
  Crmdr/1(Crmdr) -> Sum/7  "Crmdr"
  Crmblg/1(Crmblg) -> Sum/6  "Crmblg"
  Crmbdle/1(Crmbdle) -> Sum/5  "Crmbdle"
  Crmbdn/1(Crmbdn) -> Sum/4  "Crmbdn"
  Crmbde/1(Crmbde) -> Sum/3  "Crmbde"
  Crmbeta/1(Crmbeta) -> Sum/2  "Crmbeta"
  Crmbasic/1(Crmbasic) -> Sum/1  "Crmbasic"
  eoeff1/1(eoeff) -> Bus Creator/2  "eoeff"
  Bus Creator/1 -> Crmr/1(in_bus), Crmrbeta/1(in_bus), Crmrde/1(in_bus), Crmpbeta/1(in_bus), Crmp/1(in_bus), Crmbetad/1(in_bus), Crmdna/1(in_bus), Crmdayb/1(in_bus), Crmday/1(in_bus), Crmdaib/1(in_bus), Crmdai/1(in_bus), Crmdr/1(in_bus), Crmblg/1(in_bus), Crmbdle/1(in_bus), Crmbdn/1(in_bus), Crmbde/1(in_bus), Crmbeta/1(in_bus), Crmbasic/1(in_bus)  "in_bus"
  AeroIn_Bus/1 -> eoeff1/1(AeroIn_Bus), Bus Creator/1
  eoeff1/2(eieff) -> Bus Creator/3  "eieff"
  Sum/1 -> crmtot/1

== system kamerol/Aerodynamics/RollMomentCoefficient/MachRegion2 ==
  note: 0.4 < Mach < 0.5
  AeroIn_Bus : Inport
  Bus Creator : BusCreator  Inputs=3
  Crmbasic : Subsystem
  Crmbde : Subsystem
  Crmbdle : Subsystem
  Crmbdn : Subsystem
  Crmbeta : Subsystem
  Crmbetad : Subsystem
  Crmblg : Subsystem
  Crmdai : Subsystem
  Crmdaib : Subsystem
  Crmday : Subsystem
  Crmdayb : Subsystem
  Crmdna : Subsystem
  Crmdr : Subsystem
  Crmp : Subsystem
  Crmpbeta : Subsystem
  Crmr : Subsystem
  Crmrbeta : Subsystem
  Crmrde : Subsystem
  Sum : Sum  Inputs=18
  eoeff1 : Subsystem
  crmtot : Outport
  wires:
  Crmpbeta/1(Crmpbeta) -> Sum/15  "Crmpbeta"
  Crmdaib/1(Crmdaib) -> Sum/9  "Crmdaib"
  Crmdai/1(Crmdai) -> Sum/8  "Crmdai"
  Crmbasic/1(Crmbasic) -> Sum/1  "Crmbasic"
  Crmrbeta/1(Crmrbeta) -> Sum/17  "Crmrbeta"
  Crmr/1(Crmr) -> Sum/16  "Crmr"
  Crmdna/1(Crmdna) -> Sum/12  "Crmdna"
  Sum/1 -> crmtot/1
  Crmbetad/1(Crmbetad) -> Sum/13  "Crmbetad"
  Crmp/1(Crmp) -> Sum/14  "Crmp"
  AeroIn_Bus/1 -> eoeff1/1(AeroIn_Bus), Bus Creator/1
  Crmdayb/1(Crmdayb) -> Sum/11  "Crmdayb"
  eoeff1/2(eieff) -> Bus Creator/3  "eieff"
  Crmdr/1(Crmdr) -> Sum/7  "Crmdr"
  Crmbdn/1(Crmbdn) -> Sum/4  "Crmbdn"
  Crmbde/1(Crmbde) -> Sum/3  "Crmbde"
  eoeff1/1(eoeff) -> Bus Creator/2  "eoeff"
  Bus Creator/1 -> Crmr/1(in_bus), Crmrbeta/1(in_bus), Crmrde/1(in_bus), Crmpbeta/1(in_bus), Crmp/1(in_bus), Crmbetad/1(in_bus), Crmdna/1(in_bus), Crmdayb/1(in_bus), Crmday/1(in_bus), Crmdaib/1(in_bus), Crmdai/1(in_bus), Crmdr/1(in_bus), Crmblg/1(in_bus), Crmbdle/1(in_bus), Crmbdn/1(in_bus), Crmbde/1(in_bus), Crmbeta/1(in_bus), Crmbasic/1(in_bus)  "in_bus"
  Crmbdle/1(Crmbdle) -> Sum/5  "Crmbdle"
  Crmday/1(Crmday) -> Sum/10  "Crmday"
  Crmblg/1(Crmblg) -> Sum/6  "Crmblg"
  Crmbeta/1(Crmbeta) -> Sum/2  "Crmbeta"
  Crmrde/1(Crmrde) -> Sum/18  "Crmrde"

== system kamerol/Aerodynamics/RollMomentCoefficient/MachRegion3 ==
  note: 0.5 <= Mach <= 1.4
  AeroIn_Bus : Inport
  Bus Creator : BusCreator  Inputs=3
  Crmbasic : Subsystem
  Crmbde : Subsystem
  Crmbdle : Subsystem
  Crmbdn : Subsystem
  Crmbeta : Subsystem
  Crmbetad : Subsystem
  Crmblg : Subsystem
  Crmdai : Subsystem
  Crmdaib : Subsystem
  Crmday : Subsystem
  Crmdayb : Subsystem
  Crmdna : Subsystem
  Crmdr : Subsystem
  Crmp : Subsystem
  Crmpbeta : Subsystem
  Crmr : Subsystem
  Crmrbeta : Subsystem
  Crmrde : Subsystem
  Sum : Sum  Inputs=18
  eoeff1 : Subsystem
  crmtot : Outport
  wires:
  Sum/1 -> crmtot/1
  Crmrde/1(Crmrde) -> Sum/18  "Crmrde"
  Crmrbeta/1(Crmrbeta) -> Sum/17  "Crmrbeta"
  Crmr/1(Crmr) -> Sum/16  "Crmr"
  Crmpbeta/1(Crmpbeta) -> Sum/15  "Crmpbeta"
  Crmp/1(Crmp) -> Sum/14  "Crmp"
  Crmbetad/1(Crmbetad) -> Sum/13  "Crmbetad"
  Crmdna/1(Crmdna) -> Sum/12  "Crmdna"
  Crmdayb/1(Crmdayb) -> Sum/11  "Crmdayb"
  Crmday/1(Crmday) -> Sum/10  "Crmday"
  Crmdaib/1(Crmdaib) -> Sum/9  "Crmdaib"
  Crmdai/1(Crmdai) -> Sum/8  "Crmdai"
  Crmdr/1(Crmdr) -> Sum/7  "Crmdr"
  Crmblg/1(Crmblg) -> Sum/6  "Crmblg"
  Crmbdle/1(Crmbdle) -> Sum/5  "Crmbdle"
  Crmbdn/1(Crmbdn) -> Sum/4  "Crmbdn"
  Crmbde/1(Crmbde) -> Sum/3  "Crmbde"
  Crmbeta/1(Crmbeta) -> Sum/2  "Crmbeta"
  Crmbasic/1(Crmbasic) -> Sum/1  "Crmbasic"
  eoeff1/2(eieff) -> Bus Creator/3  "eieff"
  eoeff1/1(eoeff) -> Bus Creator/2  "eoeff"
  Bus Creator/1 -> Crmr/1(in_bus), Crmrde/1(in_bus), Crmp/1(in_bus), Crmbetad/1(in_bus), Crmdna/1(in_bus), Crmday/1(in_bus), Crmdai/1(in_bus), Crmdr/1(in_bus), Crmblg/1(in_bus), Crmbdle/1(in_bus), Crmbdn/1(in_bus), Crmbde/1(in_bus), Crmbeta/1(in_bus)  "in_bus"
  AeroIn_Bus/1 -> eoeff1/1(AeroIn_Bus), Bus Creator/1

== system kamerol/Aerodynamics/RollMomentCoefficient/MachRegion4 ==
  note: 1.4 < Mach
  AeroIn_Bus : Inport
  Bus Creator : BusCreator  Inputs=3
  Crmbasic : Subsystem
  Crmbde : Subsystem
  Crmbdle : Subsystem
  Crmbdn : Subsystem
  Crmbeta : Subsystem
  Crmbetad : Subsystem
  Crmblg : Subsystem
  Crmdai : Subsystem
  Crmdaib : Subsystem
  Crmday : Subsystem
  Crmdayb : Subsystem
  Crmdna : Subsystem
  Crmdr : Subsystem
  Crmp : Subsystem
  Crmpbeta : Subsystem
  Crmr : Subsystem
  Crmrbeta : Subsystem
  Crmrde : Subsystem
  Sum : Sum  Inputs=18
  eoeff1 : Subsystem
  crmtot : Outport
  wires:
  Crmrde/1(Crmrde) -> Sum/18  "Crmrde"
  Crmrbeta/1(Crmrbeta) -> Sum/17  "Crmrbeta"
  Crmr/1(Crmr) -> Sum/16  "Crmr"
  Crmpbeta/1(Crmpbeta) -> Sum/15  "Crmpbeta"
  Crmp/1(Crmp) -> Sum/14  "Crmp"
  Crmbetad/1(Crmbetad) -> Sum/13  "Crmbetad"
  Crmdna/1(Crmdna) -> Sum/12  "Crmdna"
  Crmdayb/1(Crmdayb) -> Sum/11  "Crmdayb"
  Crmday/1(Crmday) -> Sum/10  "Crmday"
  Crmdaib/1(Crmdaib) -> Sum/9  "Crmdaib"
  Crmdai/1(Crmdai) -> Sum/8  "Crmdai"
  Crmdr/1(Crmdr) -> Sum/7  "Crmdr"
  Crmblg/1(Crmblg) -> Sum/6  "Crmblg"
  Crmbdle/1(Crmbdle) -> Sum/5  "Crmbdle"
  Crmbdn/1(Crmbdn) -> Sum/4  "Crmbdn"
  Crmbde/1(Crmbde) -> Sum/3  "Crmbde"
  Crmbeta/1(Crmbeta) -> Sum/2  "Crmbeta"
  Crmbasic/1(Crmbasic) -> Sum/1  "Crmbasic"
  eoeff1/1(eoeff) -> Bus Creator/2  "eoeff"
  AeroIn_Bus/1 -> eoeff1/1(AeroIn_Bus), Bus Creator/1
  Bus Creator/1 -> Crmr/1(in_bus), Crmrde/1(in_bus), Crmp/1(in_bus), Crmbetad/1(in_bus), Crmdna/1(in_bus), Crmday/1(in_bus), Crmdai/1(in_bus), Crmdr/1(in_bus), Crmblg/1(in_bus), Crmbdle/1(in_bus), Crmbdn/1(in_bus), Crmbde/1(in_bus), Crmbeta/1(in_bus)  "in_bus"
  eoeff1/2(eieff) -> Bus Creator/3  "eieff"
  Sum/1 -> crmtot/1

== system kamerol/Aerodynamics/RollMomentCoefficient/Subsystem ==
  mach_nd : Inport
  CrmtotMR1 : Inport  Port=2
  CrmtotMR2 : Inport  Port=3
  CrmtotMR3 : Inport  Port=4
  CrmtotMR4 : Inport  Port=5
  AND : Logic  IconShape=distinctive  AllPortsSameDT=off  OutDataTypeStr=boolean
  AND1 : Logic  IconShape=distinctive  AllPortsSameDT=off  OutDataTypeStr=boolean
  Compare To Constant1 : simulink/Logic and Bit Operations/Compare To Constant  relop=<=  const=0.4  OutDataTypeStr=boolean
  Compare To Constant2 : simulink/Logic and Bit Operations/Compare To Constant  relop=>  const=0.4  OutDataTypeStr=boolean
  Compare To Constant3 : simulink/Logic and Bit Operations/Compare To Constant  relop=<  const=0.5  OutDataTypeStr=boolean
  Compare To Constant4 : simulink/Logic and Bit Operations/Compare To Constant  relop=<=  const=1.4  OutDataTypeStr=boolean
  Compare To Constant5 : simulink/Logic and Bit Operations/Compare To Constant  relop=>=  const=0.5  OutDataTypeStr=boolean
  Switch : Switch  Criteria=u2 ~= 0
  Switch1 : Switch  Criteria=u2 ~= 0
  Switch2 : Switch  Criteria=u2 ~= 0
  Crmtot : Outport
  wires:
  Compare To Constant5/1 -> AND1/1
  Compare To Constant4/1 -> AND1/2
  AND1/1 -> Switch2/2
  CrmtotMR4/1 -> Switch2/3
  CrmtotMR3/1 -> Switch2/1
  Switch/1 -> Crmtot/1
  Switch2/1 -> Switch1/3
  CrmtotMR2/1 -> Switch1/1
  Switch1/1 -> Switch/3
  CrmtotMR1/1 -> Switch/1
  AND/1 -> Switch1/2
  Compare To Constant3/1 -> AND/2
  Compare To Constant2/1 -> AND/1
  Compare To Constant1/1 -> Switch/2
  mach_nd/1 -> Compare To Constant1/1, Compare To Constant3/1, Compare To Constant4/1, Compare To Constant5/1, Compare To Constant2/1
